simulink model "HAE"  (R2018a)
(part 2 of 5)

      |         set_param(gcb,'B','0');
      |     case 'IEEE Moderately Inverse'
      |         set_param(gcb,'k','0.0515');
      |         set_param(gcb,'alpha','0.02');
      |         set_param(gcb,'B','0.114');
      |     case 'IEEE Very Inverse'
      |         set_param(gcb,'k','19.61');
      |         set_param(gcb,'alpha','2');
      |         set_param(gcb,'B','0.491');
      |     case 'IEEE Extremely Inverse'
      |         set_param(gcb,'k','28.2');
      |         set_param(gcb,'alpha','2');
      |         set_param(gcb,'B','0.1217');
      | end
      mask DialogControl Container4 Prompt: Parametros Relee
      mask DialogControl Container13 Prompt: Proteccion 50
      mask DialogControl Container14 Prompt: Proteccion 51
      mask DialogControl Plotearcurva Prompt: Curva
      mask DialogControl Plotearcurva Callback:
      | % Plotting IDMT Curve
      | close
      | TMS = str2num(get_param(gcb,'TMS1'));
      | Vp = str2num(get_param(gcb,'Vp'));
      | PS=str2num(get_param(gcb,'PS1'));
      | k = str2num(get_param(gcb,'k'));
      | alpha = str2num(get_param(gcb,'alpha'));
      | B = str2num(get_param(gcb,'B'));
      | Esc = str2num(get_param(gcb,'Esc'));
      | Tins = str2num(get_param(gcb,'Tins'));
      | I = [1.1:0.1:Esc];
      | I1=[Esc,Esc:0.1:30]
      | y=((k./((I.^alpha)-1))+B)*TMS;
      | Tin=[((k./((Esc.^alpha)-1))+B)*TMS,ones(1,length(I1)-1)*Tins];
      | loglog(I,y,'b');
      | hold on
      | loglog(I1,Tin,'b');
      | set(gcf, 'Position', [200 150 300 500]);
      | switch(get_param(gcb,'tcpopup'))
      |     case 'IEC Standard Inverse'
      |         title('IEC Standard Inverse');
      |     case 'IEC Very Inverse'
      |         title('IEC Very Inverse');
      |     case 'IEC Long Time Inverse'
      |         title('IEC Long Time Inverse');
      |     case 'IEC Extremely Inverse'
      |         title('IEC Extremely Inverse');
      |      case 'IEC Ultra Inverse'
      |         title('IEC Ultra Inverse');
      |     case 'IEEE Moderately Inverse'
      |         title('IEEE Moderately Inverse');
      |     case 'IEEE Very Inverse'
      |         title('IEEE Very Inverse');
      |     case 'IEEE Extremely Inverse'
      |         title('IEEE Extremely Inverse');
      | end
      | ymax=10^ceil(log10(max(y)));
      | set(gca, 'XTick',[1:10 20]);
      | set(gca, 'YTick',[0 ymax/1000 ymax/500 ymax/200 ymax/100 ymax/50 ymax/20 ymax/10 ymax/5 ymax/2 ymax]);
      | xlim([0.9 30]);
      | ylim([0.01 ymax]);
      | xlabel(['Corriente multiplicada por Ipick-up(' num2str(PS*Vp) 'A)']);
      | ylabel('Operating Time (sec)');
      | grid on;
      mask DialogControl Container10 Prompt: Caracteristicas Trafo Corriente
      mask Display: disp('(50/51)');
  Subsystem4 : Subsystem
      mask Display: disp('P.C.C.')
  Subsystem6 : Subsystem  mask{tcpopup=IEC Standard Inverse, k=0.14, alpha=0.02, B=0, PS1=0.834, TMS1=0.050, Tins=0.109, Esc=19, Vp=300, Vs=5, F=60}
      mask prompts: tcpopup "Disparo"; PS1 "Plug Setting (PS)/Low-set(I>)"; TMS1 "Multiplicador Tiempo"; Esc "Escala"; Vp "Primario CT"; Vs "Secundario CT"; F "Frecuencia"
      mask TypeOptions tcpopup: IEC Standard Inverse | IEC Very Inverse | IEC Long Time Inverse | IEC Extremely Inverse | IEC Ultra Inverse | IEEE Moderately Inverse | IEEE Very Inverse | IEEE Extremely Inverse
      mask Callback tcpopup:
      | switch(get_param(gcb,'tcpopup'))
      |     case 'IEC Standard Inverse'
      |         set_param(gcb,'k','0.14');
      |         set_param(gcb,'alpha','0.02');
      |         set_param(gcb,'B','0');
      |     case 'IEC Very Inverse'
      |         set_param(gcb,'k','13.5');
      |         set_param(gcb,'alpha','1');
      |         set_param(gcb,'B','0');
      |     case 'IEC Long Time Inverse'
      |         set_param(gcb,'k','120');
      |         set_param(gcb,'alpha','1');
      |         set_param(gcb,'B','0');
      |     case 'IEC Extremely Inverse'
      |         set_param(gcb,'k','80');
      |         set_param(gcb,'alpha','2');
      |         set_param(gcb,'B','0');
      |     case 'IEC Ultra Inverse'
      |         set_param(gcb,'k','315.2');
      |         set_param(gcb,'alpha','2.5');
      |         set_param(gcb,'B','0');
      |     case 'IEEE Moderately Inverse'
      |         set_param(gcb,'k','0.0515');
      |         set_param(gcb,'alpha','0.02');
      |         set_param(gcb,'B','0.114');
      |     case 'IEEE Very Inverse'
      |         set_param(gcb,'k','19.61');
      |         set_param(gcb,'alpha','2');
      |         set_param(gcb,'B','0.491');
      |     case 'IEEE Extremely Inverse'
      |         set_param(gcb,'k','28.2');
      |         set_param(gcb,'alpha','2');
      |         set_param(gcb,'B','0.1217');
      | end
      mask DialogControl Container4 Prompt: Parametros Relee
      mask DialogControl Container13 Prompt: Proteccion 50
      mask DialogControl Container14 Prompt: Proteccion 51
      mask DialogControl Plotearcurva Prompt: Curva
      mask DialogControl Plotearcurva Callback:
      | % Plotting IDMT Curve
      | close
      | TMS = str2num(get_param(gcb,'TMS1'));
      | Vp = str2num(get_param(gcb,'Vp'));
      | PS=str2num(get_param(gcb,'PS1'));
      | k = str2num(get_param(gcb,'k'));
      | alpha = str2num(get_param(gcb,'alpha'));
      | B = str2num(get_param(gcb,'B'));
      | Esc = str2num(get_param(gcb,'Esc'));
      | Tins = str2num(get_param(gcb,'Tins'));
      | I = [1.1:0.1:Esc];
      | I1=[Esc,Esc:0.1:30]
      | y=((k./((I.^alpha)-1))+B)*TMS;
      | Tin=[((k./((Esc.^alpha)-1))+B)*TMS,ones(1,length(I1)-1)*Tins];
      | loglog(I,y,'b');
      | hold on
      | loglog(I1,Tin,'b');
      | set(gcf, 'Position', [200 150 300 500]);
      | switch(get_param(gcb,'tcpopup'))
      |     case 'IEC Standard Inverse'
      |         title('IEC Standard Inverse');
      |     case 'IEC Very Inverse'
      |         title('IEC Very Inverse');
      |     case 'IEC Long Time Inverse'
      |         title('IEC Long Time Inverse');
      |     case 'IEC Extremely Inverse'
      |         title('IEC Extremely Inverse');
      |      case 'IEC Ultra Inverse'
      |         title('IEC Ultra Inverse');
      |     case 'IEEE Moderately Inverse'
      |         title('IEEE Moderately Inverse');
      |     case 'IEEE Very Inverse'
      |         title('IEEE Very Inverse');
      |     case 'IEEE Extremely Inverse'
      |         title('IEEE Extremely Inverse');
      | end
      | ymax=10^ceil(log10(max(y)));
      | set(gca, 'XTick',[1:10 20]);
      | set(gca, 'YTick',[0 ymax/1000 ymax/500 ymax/200 ymax/100 ymax/50 ymax/20 ymax/10 ymax/5 ymax/2 ymax]);
      | xlim([0.9 30]);
      | ylim([0.01 ymax]);
      | xlabel(['Corriente multiplicada por Ipick-up(' num2str(PS*Vp) 'A)']);
      | ylabel('Operating Time (sec)');
      | grid on;
      mask DialogControl Container10 Prompt: Caracteristicas Trafo Corriente
      mask Display: disp('(50/51)');
  Subsystem7 : Subsystem  mask{tcpopup=IEC Standard Inverse, k=0.14, alpha=0.02, B=0, PS1=0.640, TMS1=0.35, Tins=0.588, Esc=35, Vp=600, Vs=5, F=60}
      mask prompts: tcpopup "Disparo"; PS1 "Plug Setting (PS)/Low-set(I>)"; TMS1 "Multiplicador Tiempo"; Esc "Escala"; Vp "Primario CT"; Vs "Secundario CT"; F "Frecuencia"
      mask TypeOptions tcpopup: IEC Standard Inverse | IEC Very Inverse | IEC Long Time Inverse | IEC Extremely Inverse | IEC Ultra Inverse | IEEE Moderately Inverse | IEEE Very Inverse | IEEE Extremely Inverse
      mask Callback tcpopup:
      | switch(get_param(gcb,'tcpopup'))
      |     case 'IEC Standard Inverse'
      |         set_param(gcb,'k','0.14');
      |         set_param(gcb,'alpha','0.02');
      |         set_param(gcb,'B','0');
      |     case 'IEC Very Inverse'
      |         set_param(gcb,'k','13.5');
      |         set_param(gcb,'alpha','1');
      |         set_param(gcb,'B','0');
      |     case 'IEC Long Time Inverse'
      |         set_param(gcb,'k','120');
      |         set_param(gcb,'alpha','1');
      |         set_param(gcb,'B','0');
      |     case 'IEC Extremely Inverse'
      |         set_param(gcb,'k','80');
      |         set_param(gcb,'alpha','2');
      |         set_param(gcb,'B','0');
      |     case 'IEC Ultra Inverse'
      |         set_param(gcb,'k','315.2');
      |         set_param(gcb,'alpha','2.5');
      |         set_param(gcb,'B','0');
      |     case 'IEEE Moderately Inverse'
      |         set_param(gcb,'k','0.0515');
      |         set_param(gcb,'alpha','0.02');
      |         set_param(gcb,'B','0.114');
      |     case 'IEEE Very Inverse'
      |         set_param(gcb,'k','19.61');
      |         set_param(gcb,'alpha','2');
      |         set_param(gcb,'B','0.491');
      |     case 'IEEE Extremely Inverse'
      |         set_param(gcb,'k','28.2');
      |         set_param(gcb,'alpha','2');
      |         set_param(gcb,'B','0.1217');
      | end
      mask DialogControl Container4 Prompt: Parametros Relee
      mask DialogControl Container13 Prompt: Proteccion 50
      mask DialogControl Container14 Prompt: Proteccion 51
      mask DialogControl Plotearcurva Prompt: Curva
      mask DialogControl Plotearcurva Callback:
      | % Plotting IDMT Curve
      | close
      | TMS = str2num(get_param(gcb,'TMS1'));
      | Vp = str2num(get_param(gcb,'Vp'));
      | PS=str2num(get_param(gcb,'PS1'));
      | k = str2num(get_param(gcb,'k'));
      | alpha = str2num(get_param(gcb,'alpha'));
      | B = str2num(get_param(gcb,'B'));
      | Esc = str2num(get_param(gcb,'Esc'));
      | Tins = str2num(get_param(gcb,'Tins'));
      | I = [1.1:0.1:Esc];
      | I1=[Esc,Esc:0.1:30]
      | y=((k./((I.^alpha)-1))+B)*TMS;
      | Tin=[((k./((Esc.^alpha)-1))+B)*TMS,ones(1,length(I1)-1)*Tins];
      | loglog(I,y,'b');
      | hold on
      | loglog(I1,Tin,'b');
      | set(gcf, 'Position', [200 150 300 500]);
      | switch(get_param(gcb,'tcpopup'))
      |     case 'IEC Standard Inverse'
      |         title('IEC Standard Inverse');
      |     case 'IEC Very Inverse'
      |         title('IEC Very Inverse');
      |     case 'IEC Long Time Inverse'
      |         title('IEC Long Time Inverse');
      |     case 'IEC Extremely Inverse'
      |         title('IEC Extremely Inverse');
      |      case 'IEC Ultra Inverse'
      |         title('IEC Ultra Inverse');
      |     case 'IEEE Moderately Inverse'
      |         title('IEEE Moderately Inverse');
      |     case 'IEEE Very Inverse'
      |         title('IEEE Very Inverse');
      |     case 'IEEE Extremely Inverse'
      |         title('IEEE Extremely Inverse');
      | end
      | ymax=10^ceil(log10(max(y)));
      | set(gca, 'XTick',[1:10 20]);
      | set(gca, 'YTick',[0 ymax/1000 ymax/500 ymax/200 ymax/100 ymax/50 ymax/20 ymax/10 ymax/5 ymax/2 ymax]);
      | xlim([0.9 30]);
      | ylim([0.01 ymax]);
      | xlabel(['Corriente multiplicada por Ipick-up(' num2str(PS*Vp) 'A)']);
      | ylabel('Operating Time (sec)');
      | grid on;
      mask DialogControl Container10 Prompt: Caracteristicas Trafo Corriente
      mask Display: disp('(50/51)');
  Subsystem8 : Subsystem  mask{tcpopup=IEC Standard Inverse, k=0.14, alpha=0.02, B=0, PS1=0.840, TMS1=0.150, Tins=0.1, Esc=5, Vp=300, Vs=5, F=60}
      mask prompts: tcpopup "Disparo"; PS1 "Plug Setting (PS)/Low-set(I>)"; TMS1 "Multiplicador Tiempo"; Esc "Escala"; Vp "Primario CT"; Vs "Secundario CT"; F "Frecuencia"
      mask TypeOptions tcpopup: IEC Standard Inverse | IEC Very Inverse | IEC Long Time Inverse | IEC Extremely Inverse | IEC Ultra Inverse | IEEE Moderately Inverse | IEEE Very Inverse | IEEE Extremely Inverse
      mask Callback tcpopup:
      | switch(get_param(gcb,'tcpopup'))
      |     case 'IEC Standard Inverse'
      |         set_param(gcb,'k','0.14');
      |         set_param(gcb,'alpha','0.02');
      |         set_param(gcb,'B','0');
      |     case 'IEC Very Inverse'
      |         set_param(gcb,'k','13.5');
      |         set_param(gcb,'alpha','1');
      |         set_param(gcb,'B','0');
      |     case 'IEC Long Time Inverse'
      |         set_param(gcb,'k','120');
      |         set_param(gcb,'alpha','1');
      |         set_param(gcb,'B','0');
      |     case 'IEC Extremely Inverse'
      |         set_param(gcb,'k','80');
      |         set_param(gcb,'alpha','2');
      |         set_param(gcb,'B','0');
      |     case 'IEC Ultra Inverse'
      |         set_param(gcb,'k','315.2');
      |         set_param(gcb,'alpha','2.5');
      |         set_param(gcb,'B','0');
      |     case 'IEEE Moderately Inverse'
      |         set_param(gcb,'k','0.0515');
      |         set_param(gcb,'alpha','0.02');
      |         set_param(gcb,'B','0.114');
      |     case 'IEEE Very Inverse'
      |         set_param(gcb,'k','19.61');
      |         set_param(gcb,'alpha','2');
      |         set_param(gcb,'B','0.491');
      |     case 'IEEE Extremely Inverse'
      |         set_param(gcb,'k','28.2');
      |         set_param(gcb,'alpha','2');
      |         set_param(gcb,'B','0.1217');
      | end
      mask DialogControl Container4 Prompt: Parametros Relee
      mask DialogControl Container13 Prompt: Proteccion 50
      mask DialogControl Container14 Prompt: Proteccion 51
      mask DialogControl Plotearcurva Prompt: Curva
      mask DialogControl Plotearcurva Callback:
      | % Plotting IDMT Curve
      | close
      | TMS = str2num(get_param(gcb,'TMS1'));
      | Vp = str2num(get_param(gcb,'Vp'));
      | PS=str2num(get_param(gcb,'PS1'));
      | k = str2num(get_param(gcb,'k'));
      | alpha = str2num(get_param(gcb,'alpha'));
      | B = str2num(get_param(gcb,'B'));
      | Esc = str2num(get_param(gcb,'Esc'));
      | Tins = str2num(get_param(gcb,'Tins'));
      | I = [1.1:0.1:Esc];
      | I1=[Esc,Esc:0.1:30]
      | y=((k./((I.^alpha)-1))+B)*TMS;
      | Tin=[((k./((Esc.^alpha)-1))+B)*TMS,ones(1,length(I1)-1)*Tins];
      | loglog(I,y,'b');
      | hold on
      | loglog(I1,Tin,'b');
      | set(gcf, 'Position', [200 150 300 500]);
      | switch(get_param(gcb,'tcpopup'))
      |     case 'IEC Standard Inverse'
      |         title('IEC Standard Inverse');
      |     case 'IEC Very Inverse'
      |         title('IEC Very Inverse');
      |     case 'IEC Long Time Inverse'
      |         title('IEC Long Time Inverse');
      |     case 'IEC Extremely Inverse'
      |         title('IEC Extremely Inverse');
      |      case 'IEC Ultra Inverse'
      |         title('IEC Ultra Inverse');
      |     case 'IEEE Moderately Inverse'
      |         title('IEEE Moderately Inverse');
      |     case 'IEEE Very Inverse'
      |         title('IEEE Very Inverse');
      |     case 'IEEE Extremely Inverse'
      |         title('IEEE Extremely Inverse');
      | end
      | ymax=10^ceil(log10(max(y)));
      | set(gca, 'XTick',[1:10 20]);
      | set(gca, 'YTick',[0 ymax/1000 ymax/500 ymax/200 ymax/100 ymax/50 ymax/20 ymax/10 ymax/5 ymax/2 ymax]);
      | xlim([0.9 30]);
      | ylim([0.01 ymax]);
      | xlabel(['Corriente multiplicada por Ipick-up(' num2str(PS*Vp) 'A)']);
      | ylabel('Operating Time (sec)');
      | grid on;
      mask DialogControl Container10 Prompt: Caracteristicas Trafo Corriente
      mask Display: disp('(50/51)');
  Subsystem9 : Subsystem  mask{tcpopup=IEC Standard Inverse, k=0.14, alpha=0.02, B=0, PS1=1.04, TMS1=0.170, Tins=0.398, Esc=19, Vp=300, Vs=5, F=60}
      mask prompts: tcpopup "Disparo"; PS1 "Plug Setting (PS)/Low-set(I>)"; TMS1 "Multiplicador Tiempo"; Esc "Escala"; Vp "Primario CT"; Vs "Secundario CT"; F "Frecuencia"
      mask TypeOptions tcpopup: IEC Standard Inverse | IEC Very Inverse | IEC Long Time Inverse | IEC Extremely Inverse | IEC Ultra Inverse | IEEE Moderately Inverse | IEEE Very Inverse | IEEE Extremely Inverse
      mask Callback tcpopup:
      | switch(get_param(gcb,'tcpopup'))
      |     case 'IEC Standard Inverse'
      |         set_param(gcb,'k','0.14');
      |         set_param(gcb,'alpha','0.02');
      |         set_param(gcb,'B','0');
      |     case 'IEC Very Inverse'
      |         set_param(gcb,'k','13.5');
      |         set_param(gcb,'alpha','1');
      |         set_param(gcb,'B','0');
      |     case 'IEC Long Time Inverse'
      |         set_param(gcb,'k','120');
      |         set_param(gcb,'alpha','1');
      |         set_param(gcb,'B','0');
      |     case 'IEC Extremely Inverse'
      |         set_param(gcb,'k','80');
      |         set_param(gcb,'alpha','2');
      |         set_param(gcb,'B','0');
      |     case 'IEC Ultra Inverse'
      |         set_param(gcb,'k','315.2');
      |         set_param(gcb,'alpha','2.5');
      |         set_param(gcb,'B','0');
      |     case 'IEEE Moderately Inverse'
      |         set_param(gcb,'k','0.0515');
      |         set_param(gcb,'alpha','0.02');
      |         set_param(gcb,'B','0.114');
      |     case 'IEEE Very Inverse'
      |         set_param(gcb,'k','19.61');
      |         set_param(gcb,'alpha','2');
      |         set_param(gcb,'B','0.491');
      |     case 'IEEE Extremely Inverse'
      |         set_param(gcb,'k','28.2');
      |         set_param(gcb,'alpha','2');
      |         set_param(gcb,'B','0.1217');
      | end
      mask DialogControl Container4 Prompt: Parametros Relee
      mask DialogControl Container13 Prompt: Proteccion 50
      mask DialogControl Container14 Prompt: Proteccion 51
      mask DialogControl Plotearcurva Prompt: Curva
      mask DialogControl Plotearcurva Callback:
      | % Plotting IDMT Curve
      | close
      | TMS = str2num(get_param(gcb,'TMS1'));
      | Vp = str2num(get_param(gcb,'Vp'));
      | PS=str2num(get_param(gcb,'PS1'));
      | k = str2num(get_param(gcb,'k'));
      | alpha = str2num(get_param(gcb,'alpha'));
      | B = str2num(get_param(gcb,'B'));
      | Esc = str2num(get_param(gcb,'Esc'));
      | Tins = str2num(get_param(gcb,'Tins'));
      | I = [1.1:0.1:Esc];
      | I1=[Esc,Esc:0.1:30]
      | y=((k./((I.^alpha)-1))+B)*TMS;
      | Tin=[((k./((Esc.^alpha)-1))+B)*TMS,ones(1,length(I1)-1)*Tins];
      | loglog(I,y,'b');
      | hold on
      | loglog(I1,Tin,'b');
      | set(gcf, 'Position', [200 150 300 500]);
      | switch(get_param(gcb,'tcpopup'))
      |     case 'IEC Standard Inverse'
      |         title('IEC Standard Inverse');
      |     case 'IEC Very Inverse'
      |         title('IEC Very Inverse');
      |     case 'IEC Long Time Inverse'
      |         title('IEC Long Time Inverse');
      |     case 'IEC Extremely Inverse'
      |         title('IEC Extremely Inverse');
      |      case 'IEC Ultra Inverse'
      |         title('IEC Ultra Inverse');
      |     case 'IEEE Moderately Inverse'
      |         title('IEEE Moderately Inverse');
      |     case 'IEEE Very Inverse'
      |         title('IEEE Very Inverse');
      |     case 'IEEE Extremely Inverse'
      |         title('IEEE Extremely Inverse');
      | end
      | ymax=10^ceil(log10(max(y)));
      | set(gca, 'XTick',[1:10 20]);
      | set(gca, 'YTick',[0 ymax/1000 ymax/500 ymax/200 ymax/100 ymax/50 ymax/20 ymax/10 ymax/5 ymax/2 ymax]);
      | xlim([0.9 30]);
      | ylim([0.01 ymax]);
      | xlabel(['Corriente multiplicada por Ipick-up(' num2str(PS*Vp) 'A)']);
      | ylabel('Operating Time (sec)');
      | grid on;
      mask DialogControl Container10 Prompt: Caracteristicas Trafo Corriente
      mask Display: disp('(50/51)');
  Switch1 : Switch  Criteria=u2 ~= 0
  Switch2 : Switch  Criteria=u2 ~= 0
  T1 : powerlib/Elements/Three-Phase Transformer (Two Windings)  Winding1Connection=Delta (D11)  Winding2Connection=Yg  CoreType=Three single-phase transformers  SetSaturation=off  Hysteresis=off  DataFile='basic_model'  SetInitialFlux=off  Measurements=None  UNITS=pu  NominalPower=[60e6 60 ]  Winding1=[115e+03 0.00033931 0.010485]  Winding2=[13.8e+3 0.0057021 0.17621]  Rm=74.757  Lm=74.756  L0=0.5  Saturation=[0 0;0.01413 0.50702;2.8261 0.59153]  InitialFluxes=[0.33801 -0.33801 0.29576]  MoreParameters=off  BreakLoop=off  DataType=off  TransfoNumber=0
  T2 : powerlib/Elements/Three-Phase Transformer (Two Windings)  Winding1Connection=Delta (D11)  Winding2Connection=Yg  CoreType=Three single-phase transformers  SetSaturation=off  Hysteresis=off  DataFile='basic_model'  SetInitialFlux=off  Measurements=None  UNITS=pu  NominalPower=[60e6 60 ]  Winding1=[115e+03 0.00033931 0.010485]  Winding2=[13.8e+3 0.0057021 0.17621]  Rm=74.757  Lm=74.756  L0=0.5  Saturation=[0 0;0.01413 0.50702;2.8261 0.59153]  InitialFluxes=[0.33801 -0.33801 0.29576]  MoreParameters=off  BreakLoop=off  DataType=off  TransfoNumber=0
  T3 : powerlib/Elements/Three-Phase Transformer (Two Windings)  Winding1Connection=Delta (D11)  Winding2Connection=Yg  CoreType=Three single-phase transformers  SetSaturation=off  Hysteresis=off  DataFile='basic_model'  SetInitialFlux=off  Measurements=None  UNITS=pu  NominalPower=[40e6 60 ]  Winding1=[13.8e+03 0.00033931 0.010485]  Winding2=[0.48e+3 0.0057021 0.17621]  Rm=74.757  Lm=74.756  L0=0.5  Saturation=[0 0;0.01413 0.50702;2.8261 0.59153]  InitialFluxes=[0.33801 -0.33801 0.29576]  MoreParameters=off  BreakLoop=off  DataType=off  TransfoNumber=0
  T4 : powerlib/Elements/Three-Phase Transformer (Two Windings)  Winding1Connection=Delta (D11)  Winding2Connection=Yg  CoreType=Three single-phase transformers  SetSaturation=off  Hysteresis=off  DataFile='basic_model'  SetInitialFlux=off  Measurements=None  UNITS=pu  NominalPower=[40e6 60 ]  Winding1=[13.8e+03 0.00033931 0.010485]  Winding2=[0.48e+3 0.0057021 0.17621]  Rm=74.757  Lm=74.756  L0=0.5  Saturation=[0 0;0.01413 0.50702;2.8261 0.59153]  InitialFluxes=[0.33801 -0.33801 0.29576]  MoreParameters=off  BreakLoop=off  DataType=off  TransfoNumber=0
  TC_R10 : powerlib/Measurements/Three-Phase V-I Measurement  VoltageMeasurement=phase-to-ground  SetLabelV=on  LabelV=V_F_F10  Vpu=off  VpuLL=off  CurrentMeasurement=yes  SetLabelI=on  LabelI=TC_R10  Ipu=off  Pbase=100e6  Vbase=500e3  OutputType=Complex  PhasorSimulation=off  PSBequivalent=0
  TC_R5 : powerlib/Measurements/Three-Phase V-I Measurement  VoltageMeasurement=phase-to-ground  SetLabelV=on  LabelV=V_F_R5  Vpu=off  VpuLL=off  CurrentMeasurement=yes  SetLabelI=on  LabelI=TC_R5  Ipu=off  Pbase=100e6  Vbase=500e3  OutputType=Complex  PhasorSimulation=off  PSBequivalent=0
  TC_R6 : powerlib/Measurements/Three-Phase V-I Measurement  VoltageMeasurement=phase-to-ground  SetLabelV=on  LabelV=V_F_RM_1  Vpu=off  VpuLL=off  CurrentMeasurement=yes  SetLabelI=on  LabelI=TC_R6  Ipu=off  Pbase=100e6  Vbase=500e3  OutputType=Complex  PhasorSimulation=off  PSBequivalent=0
  TC_R7 : powerlib/Measurements/Three-Phase V-I Measurement  VoltageMeasurement=phase-to-ground  SetLabelV=on  LabelV=V_F_L7  Vpu=off  VpuLL=off  CurrentMeasurement=yes  SetLabelI=on  LabelI=TC_R7  Ipu=off  Pbase=100e6  Vbase=500e3  OutputType=Complex  PhasorSimulation=off  PSBequivalent=0
  TC_R8 : powerlib/Measurements/Three-Phase V-I Measurement  VoltageMeasurement=phase-to-ground  SetLabelV=on  LabelV=V_F_8  Vpu=off  VpuLL=off  CurrentMeasurement=yes  SetLabelI=on  LabelI=TC_R8  Ipu=off  Pbase=100e6  Vbase=500e3  OutputType=Complex  PhasorSimulation=off  PSBequivalent=0
  TC_R9 : powerlib/Measurements/Three-Phase V-I Measurement  VoltageMeasurement=phase-to-ground  SetLabelV=on  LabelV=V_F_R9  Vpu=off  VpuLL=off  CurrentMeasurement=yes  SetLabelI=on  LabelI=TC_R9  Ipu=off  Pbase=100e6  Vbase=500e3  OutputType=Complex  PhasorSimulation=off  PSBequivalent=0
  Three-Phase PI Section Line2 : powerlib/Elements/Three-Phase PI Section Line  LConnTagsString=a|b|c  RConnTagsString=A|B|C  Frequency=60  Resistances=[ 0.292 0.292/2]  Inductances="[0.00094  0.00094/2]"  Capacitances=[12.74e-9 7.751e-9]  Length=1
      settings: SourceProductName=Simscape Power Systems
  Three-Phase PI Section Line3 : powerlib/Elements/Three-Phase PI Section Line  LConnTagsString=a|b|c  RConnTagsString=A|B|C  Frequency=60  Resistances=[ 0.292 0.292/2]  Inductances="[0.00094  0.00094/2]"  Capacitances=[12.74e-9 7.751e-9]  Length=0.8
      settings: SourceProductName=Simscape Power Systems
  Three-Phase PI Section Line4 : powerlib/Elements/Three-Phase PI Section Line  LConnTagsString=a|b|c  RConnTagsString=A|B|C  Frequency=60  Resistances=[ 0.292 0.292/2]  Inductances="[0.00094  0.00094/2]"  Capacitances=[12.74e-9 7.751e-9]  Length=0.8
      settings: SourceProductName=Simscape Power Systems
  Three-Phase PI Section Line6 : powerlib/Elements/Three-Phase PI Section Line  LConnTagsString=a|b|c  RConnTagsString=A|B|C  Frequency=60  Resistances=[ 0.292 0.292/2]  Inductances="[0.00094  0.00094/2]"  Capacitances=[12.74e-9 7.751e-9]  Length=1
      settings: SourceProductName=Simscape Power Systems
  Three-Phase Fault1 : powerlib/Elements/Three-Phase Fault  InitialStates=0  FaultA=on  FaultB=on  FaultC=on  GroundFault=on  SwitchTimes=1.3  External=off  SwitchStatus=NaN  FaultResistance=0.2  GroundResistance=2  SnubberResistance=1e6  SnubberCapacitance=inf  Measurements=None
  powergui : powerlib/powergui  Priority=1  SimulationMode=Discrete  SampleTime=Ts  frequency=60  Iterations=50  frequencyindice=0  Pbase=100e6  ErrMax=1e-4  UnitsV=kV  UnitsW=MW  buscounter=0  FunctionMessages=off  echomessages=off  EnableUseOfTLC=off  CurrentSourceSwitches=off  DisableSnubberDevices=off  DisableRonSwitches=off  DisableVfSwitches=off  DisplayEquations=off  SolverType=Tustin/Backward Euler (TBE)  Interpol=off  ExternalGateDelay=off  methode=off  Ts=10  x0status=blocks  SPID=off  SwTol=0  HookPort=off  RestoreLinks=warning  ResistiveCurrentMeasurement=off  Frange=[0:2:500]  Ylog=off  Xlog=on  ShowGrid=off  save=off  variable=ZData  structure=0  ZoomFFT=off  StartTime=0.0  cycles=1  DisplayStyle=1  fundamental=60  FreqAxis=off  MaxFrequency=1000  frequencyindicesteady=1  RmsSteady=1  display=off
  wires:
  [TC_R5] -> Subsystem9/1(I)
  [TC_R9] -> Subsystem10/1(I)
  [TC_R2] -> Subsystem1/1(I)
  Subsystem1/1(Trip) -> R2/1
  [TC_R1] -> Subsystem6/1(I)
  [TC_R4] -> RB1/2(I)
  [TC_R3] -> Subsystem3/1(I)
  [TC_R8] -> RB4/2(I)
  [TC_R6] -> Subsystem8/1(I)
  Subsystem3/1(Trip) -> R3/1
  Subsystem7/1(Trip) -> R7/1
  Subsystem8/1(Trip) -> R6/1
  Subsystem10/1(Trip) -> R9/1
  Subsystem9/1(Trip) -> R5/1
  Subsystem6/1(Trip) -> R1/1
  [TC_R7] -> Subsystem7/1(I)
  [TC_R10] -> RB5/2(I)
  [Config] -> RB4/1(En)
  [Config] -> RB5/1(En)
  [Config] -> RB1/1(En)
  RB1/1(Trip) -> R4/1, [DR4]
  RB4/1(Trip) -> [DR8], R8/1
  RB5/1(Trip) -> [DR10], R10/1
  [Config_g] -> Bus B2 M1/3
  [DR10] -> Bus B2 M3/1
  [TC_R4] -> Subsystem/1, Bus B2 M1/2
  [DR4] -> Bus B2 M3/3
  Subsystem/1 -> Bus B2 M1/1
  [DR8] -> Bus B2 M3/2
  Demux/2 -> Switch2/1, Switch2/2
  Demux/1 -> Switch1/1, Switch1/2
  Configuración inicial2/1 -> Switch2/3
  Configuración inicial1/1 -> Switch1/3
  Switch1/1 -> [Config], Display/1
  Switch2/1 -> Display3/1, [Config_g]
  Articulo 2 1/1(Trip) -> [te]
  [te] -> EMISOR-RECEPTOR/1(In1)
  EMISOR-RECEPTOR/1(Out1) -> Demux/1
  connections:
  P2/RConn1 -- TC_R5/LConn1 -- TC_R6/LConn1
  P3/RConn2 -- TC_R8/LConn2 -- TC_R7/LConn2
  P3/RConn1 -- TC_R7/LConn1 -- TC_R8/LConn1
  TC_R5/LConn2 -- TC_R6/LConn2 -- P2/RConn2
  P2/RConn3 -- TC_R5/LConn3 -- TC_R6/LConn3
  TC_R9/LConn1 -- P1 115 kV/RConn1 -- TC_R10/LConn1
  TC_R9/LConn2 -- TC_R10/LConn2 -- P1 115 kV/RConn2
  P3/RConn3 -- TC_R7/LConn3 -- TC_R8/LConn3
  R9/RConn2 -- T1/LConn2
  R9/RConn1 -- T1/LConn1
  TC_R9/RConn1 -- R9/LConn1
  TC_R9/RConn2 -- R9/LConn2
  R9/RConn3 -- T1/LConn3
  TC_R9/RConn3 -- R9/LConn3
  R10/RConn2 -- T2/LConn2
  R10/RConn1 -- T2/LConn1
  R10/RConn3 -- T2/LConn3
  TC_R9/LConn3 -- P1 115 kV/RConn3 -- TC_R10/LConn3
  Subsystem4/RConn1 -- P1 115 kV/LConn1
  Subsystem4/RConn2 -- P1 115 kV/LConn2
  Subsystem4/RConn3 -- P1 115 kV/LConn3
  TC_R10/RConn1 -- R10/LConn1
  TC_R10/RConn2 -- R10/LConn2
  TC_R10/RConn3 -- R10/LConn3
  P2/LConn1 -- T1/RConn1
  P2/LConn2 -- T1/RConn2
  P2/LConn3 -- T1/RConn3
  P3/LConn1 -- T2/RConn1
  P3/LConn2 -- T2/RConn2
  P3/LConn3 -- T2/RConn3
  TC_R5/RConn1 -- R5/LConn1
  TC_R5/RConn2 -- R5/LConn2
  TC_R5/RConn3 -- R5/LConn3
  Three-Phase PI Section Line6/LConn1 -- R5/RConn1
  Three-Phase PI Section Line6/LConn2 -- R5/RConn2
  Three-Phase PI Section Line6/LConn3 -- R5/RConn3
  P4 TC_R1/LConn1 -- Three-Phase PI Section Line6/RConn1
  P4 TC_R1/RConn1 -- R1/LConn1
  P4 TC_R1/LConn2 -- Three-Phase PI Section Line6/RConn2
  P4 TC_R1/LConn3 -- Three-Phase PI Section Line6/RConn3
  P4 TC_R1/RConn2 -- R1/LConn2
  P4 TC_R1/RConn3 -- R1/LConn3
  R1/RConn1 -- Carga 1/LConn1
  R1/RConn2 -- Carga 1/LConn2
  R1/RConn3 -- Carga 1/LConn3
  TC_R6/RConn1 -- R6/LConn1
  TC_R6/RConn2 -- R6/LConn2
  TC_R6/RConn3 -- R6/LConn3
  Three-Phase PI Section Line2/LConn1 -- R6/RConn1
  R6/RConn2 -- Three-Phase PI Section Line2/LConn2
  R6/RConn3 -- Three-Phase PI Section Line2/LConn3
  R2/RConn1 -- Carga 2/LConn1
  R2/RConn2 -- Carga 2/LConn2
  R2/RConn3 -- Carga 2/LConn3
  P5 TC_R2/RConn1 -- R2/LConn1
  P5 TC_R2/LConn1 -- Three-Phase PI Section Line2/RConn1
  Three-Phase PI Section Line2/RConn2 -- P5 TC_R2/LConn2
  Three-Phase PI Section Line2/RConn3 -- P5 TC_R2/LConn3
  P5 TC_R2/RConn2 -- R2/LConn2
  P5 TC_R2/RConn3 -- R2/LConn3
  TC_R7/RConn1 -- R7/LConn1
  TC_R7/RConn2 -- R7/LConn2
  TC_R7/RConn3 -- R7/LConn3
  R7/RConn1 -- Three-Phase PI Section Line4/LConn1
  R7/RConn2 -- Three-Phase PI Section Line4/LConn2
  R7/RConn3 -- Three-Phase PI Section Line4/LConn3
  P6 TC_R3/LConn1 -- Three-Phase PI Section Line4/RConn1
  P6 TC_R3/RConn1 -- R3/LConn1
  Three-Phase PI Section Line4/RConn2 -- P6 TC_R3/LConn2
  Three-Phase PI Section Line4/RConn3 -- P6 TC_R3/LConn3
  P6 TC_R3/RConn2 -- R3/LConn2
  P6 TC_R3/RConn3 -- R3/LConn3
  T3/LConn1 -- R3/RConn1
  T3/LConn2 -- R3/RConn2
  T3/LConn3 -- R3/RConn3
  Carga 3/LConn1 -- T3/RConn1
  Carga 3/LConn2 -- T3/RConn2
  Carga 3/LConn3 -- T3/RConn3
  TC_R8/RConn1 -- R8/LConn1
  TC_R8/RConn2 -- R8/LConn2
  TC_R8/RConn3 -- R8/LConn3
  Three-Phase PI Section Line3/LConn1 -- R8/RConn1
  Three-Phase PI Section Line3/LConn2 -- R8/RConn2
  Three-Phase PI Section Line3/LConn3 -- R8/RConn3
  P7 TC_R4/LConn1 -- Three-Phase PI Section Line3/RConn1
  P7 TC_R4/LConn2 -- Three-Phase PI Section Line3/RConn2
  P7 TC_R4/LConn3 -- Three-Phase PI Section Line3/RConn3
  R4/LConn1 -- P7 TC_R4/RConn1
  R4/LConn2 -- P7 TC_R4/RConn2
  R4/LConn3 -- P7 TC_R4/RConn3
  R4/RConn1 -- Three-Phase Fault1/LConn1 -- T4/LConn1
  R4/RConn2 -- Three-Phase Fault1/LConn2 -- T4/LConn2
  R4/RConn3 -- Three-Phase Fault1/LConn3 -- T4/LConn3
  Articulo 2 1/LConn1 -- T4/RConn1
  Articulo 2 1/LConn2 -- T4/RConn2
  Articulo 2 1/LConn3 -- T4/RConn3
